simulink subsystem "ControladorAJ"  (R2023b)
settings: Solver=VariableStepAuto  StartTime=0.0  StopTime=10.0  RelTol=1e-3
settings Model: Creator=USUARIO  LastModifiedBy=USUARIO

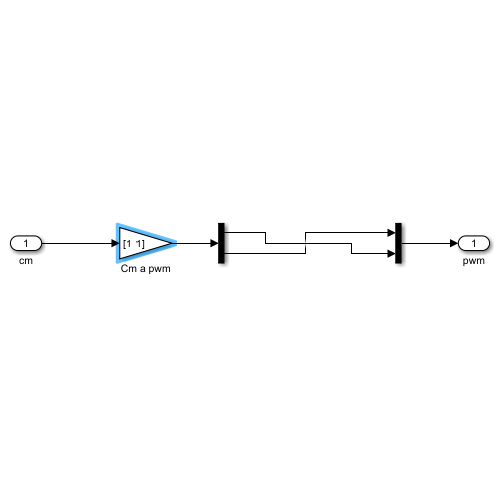
[thumbnail: Simulink's stored preview of the top-level diagram]
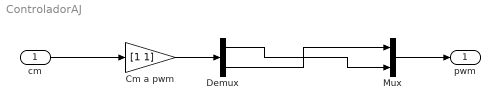
== system ControladorAJ ==
  cm : Inport
  Cm a pwm : Gain  Gain=[1 1]  OutDataTypeStr=int16
  Demux : Demux  Outputs=2
  Mux : Mux  Inputs=2
  pwm : Outport
  wires:
  Demux/2 -> Mux/1
  Demux/1 -> Mux/2
  Mux/1 -> pwm/1
  cm/1 -> Cm a pwm/1
  Cm a pwm/1 -> Demux/1
